simulink model "UUV_System"  (R2016a)
settings: Solver=VariableStepAuto  StartTime=0.0  StopTime=100  RelTol=1e-3
settings Model: Creator=Administrator  LastModifiedBy=Administrator

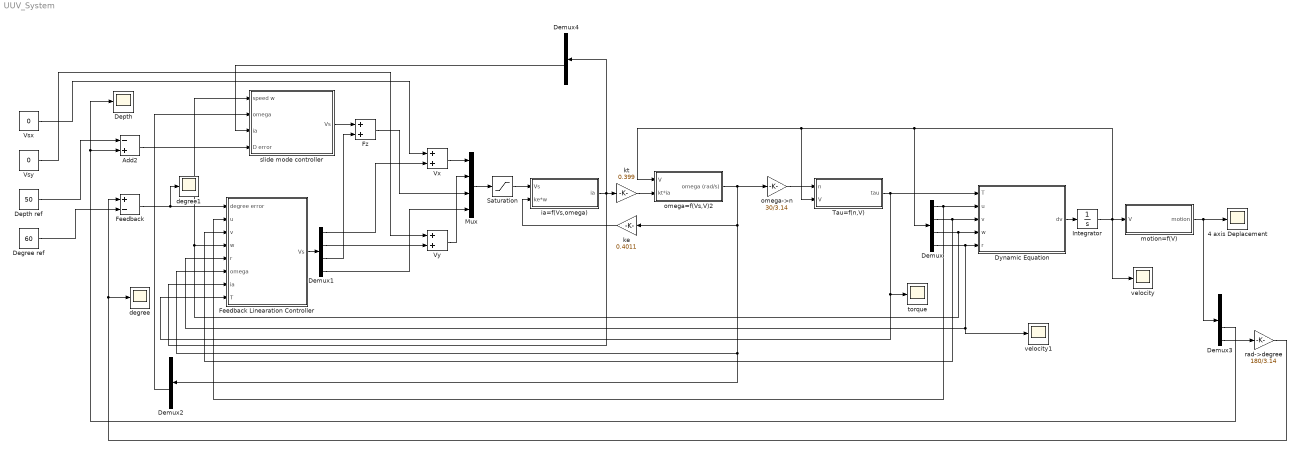
== system UUV_System ==
  "4 axis Deplacement " : Scope
  Add2 : Sum  Inputs=-+
  Degree ref : Constant  Value=60
  Demux{,1..4} (5 alike) : Demux
  Depth : Scope
  Depth ref : Constant  Value=50
  Dynamic Equation : MATLAB Function  TreatAsAtomicUnit=on
  Feedback : Sum  Inputs=+-
  Feedback Linearation Controller : Subsystem
  Fz : Sum
  Integrator : Integrator
  Mux : Mux
  Saturation : Saturate  UpperLimit=100  LowerLimit=-100
  Tau=f(n,V) : Subsystem
  Vsx : Constant  Value=0
  Vsy : Constant  Value=0
  Vx : Sum
  Vy : Sum
  degree : Scope
  degree1 : Scope
  ia=f(Vs,omega) : Subsystem
  ke : Gain  Gain=0.4011
  kt : Gain  Gain=0.399
  motion=f(V) : Subsystem
  omega->n : Gain  Gain=30/3.14
  omega=f(Vs,V)2 : Subsystem
  rad->degree : Gain  Gain=180/3.14
  slide mode controller : Subsystem
  torque : Scope
  velocity : Scope
  velocity1 : Scope
  wires:
  ia=f(Vs,omega)/1(ia) -> Feedback Linearation Controller/7(ia), Demux4/1, kt/1
  kt/1 -> omega=f(Vs,V)2/2(kt*ia)
  omega=f(Vs,V)2/1(omega (rad/s)) -> omega->n/1, Feedback Linearation Controller/6(omega), Demux2/1, ke/1
  ke/1 -> ia=f(Vs,omega)/2(ke*w)
  omega->n/1 -> Tau=f(n,V)/1(n)
  Tau=f(n,V)/1(tau) -> Dynamic Equation/1(T), Feedback Linearation Controller/8(T), torque/1
  Dynamic Equation/1(dv) -> Integrator/1
  Integrator/1 -> motion=f(V)/1(V), Demux/1, Tau=f(n,V)/2(V), omega=f(Vs,V)2/1(V), velocity/1
  Demux/1 -> Feedback Linearation Controller/2(u), Dynamic Equation/2(u)
  Demux/2 -> Feedback Linearation Controller/3(v), Dynamic Equation/3(v)
  Demux/3 -> Dynamic Equation/4(w), slide mode controller/1(speed w), Feedback Linearation Controller/4(w)
  Demux/4 -> velocity1/1, Feedback Linearation Controller/5(r), Dynamic Equation/5(r)
  motion=f(V)/1(motion) -> "4 axis Deplacement "/1, Demux3/1
  Demux1/4 -> Mux/4
  slide mode controller/1(Vs) -> Fz/1
  Demux1/3 -> Fz/2
  Fz/1 -> Mux/3
  Demux1/2 -> Vy/2
  Demux1/1 -> Vx/2
  Vx/1 -> Mux/1
  Vy/1 -> Mux/2
  Demux2/3 -> slide mode controller/2(omega)
  Degree ref/1 -> Feedback/2
  Feedback/1 -> degree1/1, Feedback Linearation Controller/1(degree error)
  Demux4/3 -> slide mode controller/3(ia)
  Depth ref/1 -> Add2/1
  Add2/1 -> slide mode controller/4(D error)
  Demux3/3 -> Depth/1, Add2/2
  Vsx/1 -> Vx/1
  Vsy/1 -> Vy/1
  Mux/1 -> Saturation/1
  Saturation/1 -> ia=f(Vs,omega)/1(Vs)
  Demux3/4 -> rad->degree/1
  rad->degree/1 -> degree/1, Feedback/1
  Feedback Linearation Controller/1(Vs) -> Demux1/1

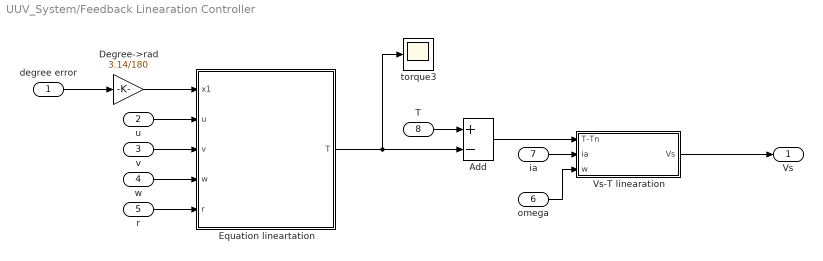
== system UUV_System/Feedback Linearation Controller ==
  degree error : Inport
  u : Inport  Port=2
  v : Inport  Port=3
  w : Inport  Port=4
  r : Inport  Port=5
  omega : Inport  Port=6
  ia : Inport  Port=7
  T : Inport  Port=8
  Add : Sum  Inputs=+-
  Degree->rad : Gain  Gain=3.14/180
  Equation lineartation : MATLAB Function  TreatAsAtomicUnit=on
  Vs-T linearation : Subsystem
  torque3 : Scope
  Vs : Outport
  wires:
  Vs-T linearation/1(Vs) -> Vs/1
  Add/1 -> Vs-T linearation/1(T-Tn)
  Equation lineartation/1(T) -> torque3/1, Add/2
  ia/1 -> Vs-T linearation/2(ia)
  omega/1 -> Vs-T linearation/3(w)
  T/1 -> Add/1
  u/1 -> Equation lineartation/2(u)
  r/1 -> Equation lineartation/5(r)
  w/1 -> Equation lineartation/4(w)
  v/1 -> Equation lineartation/3(v)
  Degree->rad/1 -> Equation lineartation/1(x1)
  degree error/1 -> Degree->rad/1

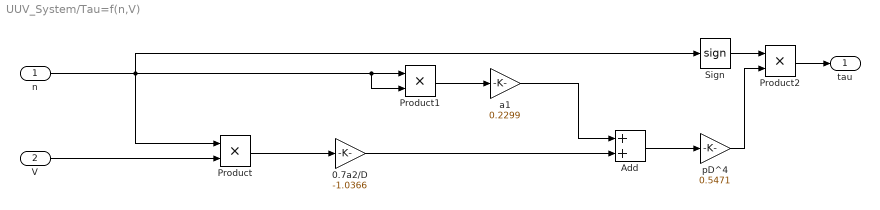
== system UUV_System/Tau=f(n,V) ==
  n : Inport
  V : Inport  Port=2
  0.7a2/D : Gain  Gain=-1.0366
  Add : Sum
  Product : Product
  Product1 : Product
  Product2 : Product
  Sign : Signum
  a1 : Gain  Gain=0.2299
  pD^4 : Gain  Gain=0.5471
  tau : Outport
  wires:
  n/1 -> Sign/1, Product/1, Product1/2, Product1/1
  V/1 -> Product/2
  Product1/1 -> a1/1
  Product/1 -> 0.7a2/D/1
  a1/1 -> Add/1
  0.7a2/D/1 -> Add/2
  Add/1 -> pD^4/1
  Sign/1 -> Product2/1
  pD^4/1 -> Product2/2
  Product2/1 -> tau/1

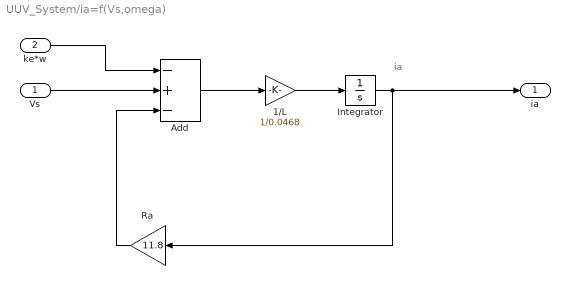
== system UUV_System/ia=f(Vs,omega) ==
  note: ia
  Vs : Inport
  ke*w : Inport  Port=2
  1/L : Gain  Gain=1/0.0468
  Add : Sum  Inputs=-+-
  Integrator : Integrator
  Ra : Gain  Gain=11.8
  ia : Outport
  wires:
  Add/1 -> 1/L/1
  1/L/1 -> Integrator/1
  Integrator/1 -> ia/1, Ra/1
  Ra/1 -> Add/3
  Vs/1 -> Add/2
  ke*w/1 -> Add/1

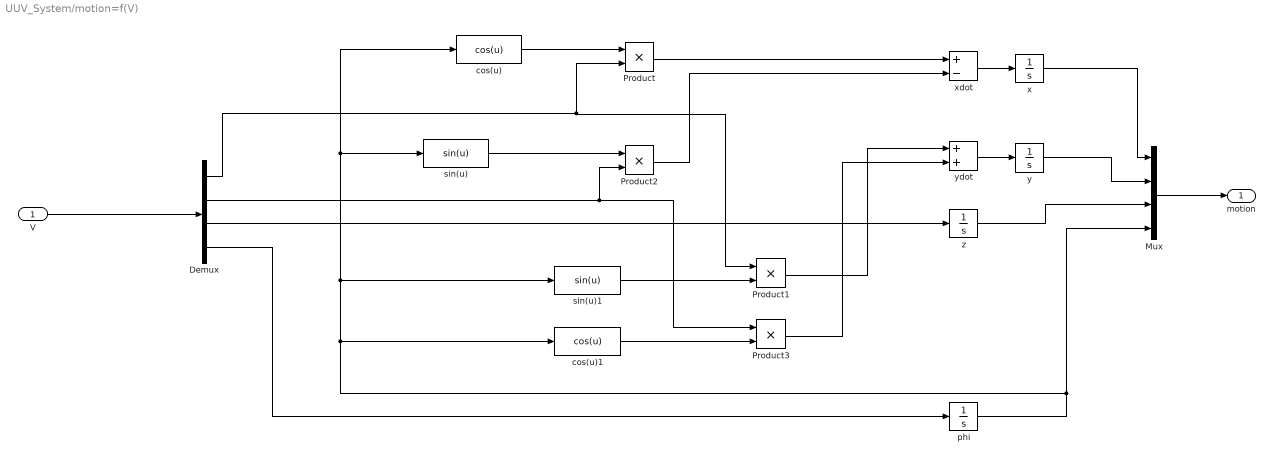
== system UUV_System/motion=f(V) ==
  V : Inport
  Demux : Demux
  Mux : Mux
  Product{,1..3} (4 alike) : Product
  cos(u) : MATLABFcn  MATLABFcn=cos(u)
  cos(u)1 : MATLABFcn  MATLABFcn=cos(u)
  phi : Integrator
  sin(u) : MATLABFcn  MATLABFcn=sin(u)
  sin(u)1 : MATLABFcn  MATLABFcn=sin(u)
  x : Integrator
  xdot : Sum  Inputs=+-
  y : Integrator
  ydot : Sum
  z : Integrator
  motion : Outport
  wires:
  V/1 -> Demux/1
  cos(u)/1 -> Product/1
  Demux/1 -> Product/2, Product1/1
  Product/1 -> xdot/1
  sin(u)/1 -> Product2/1
  Demux/2 -> Product3/1, Product2/2
  Product2/1 -> xdot/2
  sin(u)1/1 -> Product1/2
  cos(u)1/1 -> Product3/2
  Product1/1 -> ydot/1
  Product3/1 -> ydot/2
  Demux/3 -> z/1
  Demux/4 -> phi/1
  z/1 -> Mux/3
  Mux/1 -> motion/1
  phi/1 -> Mux/4, cos(u)1/1, sin(u)1/1, cos(u)/1, sin(u)/1
  xdot/1 -> x/1
  x/1 -> Mux/1
  ydot/1 -> y/1
  y/1 -> Mux/2

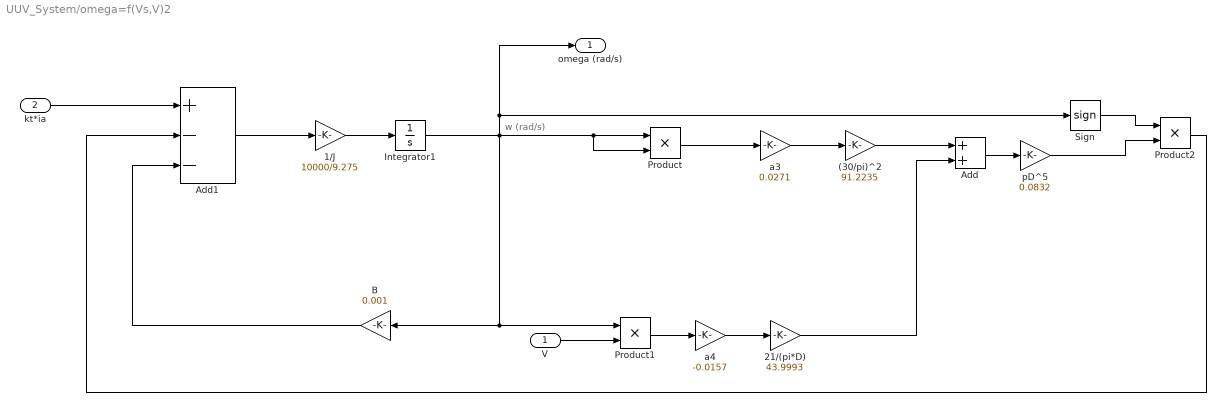
== system UUV_System/omega=f(Vs,V)2 ==
  note: w (rad/s)
  V : Inport
  kt*ia : Inport  Port=2
  (30/pi)^2 : Gain  Gain=91.2235
  1/J : Gain  Gain=10000/9.275
  21/(pi*D) : Gain  Gain=43.9993
  Add : Sum
  Add1 : Sum  Inputs=+--
  B : Gain  Gain=0.001
  Integrator1 : Integrator
  Product : Product
  Product1 : Product
  Product2 : Product
  Sign : Signum
  a3 : Gain  Gain=0.0271
  a4 : Gain  Gain=-0.0157
  pD^5 : Gain  Gain=0.0832
  omega (rad/s) : Outport
  wires:
  1/J/1 -> Integrator1/1
  Add1/1 -> 1/J/1
  B/1 -> Add1/3
  Integrator1/1 -> Product/2, Product/1, omega (rad/s)/1, Sign/1, Product1/1, B/1
  kt*ia/1 -> Add1/1
  Product/1 -> a3/1
  a3/1 -> (30/pi)^2/1
  (30/pi)^2/1 -> Add/1
  a4/1 -> 21/(pi*D)/1
  V/1 -> Product1/2
  Product1/1 -> a4/1
  21/(pi*D)/1 -> Add/2
  Add/1 -> pD^5/1
  Sign/1 -> Product2/1
  pD^5/1 -> Product2/2
  Product2/1 -> Add1/2

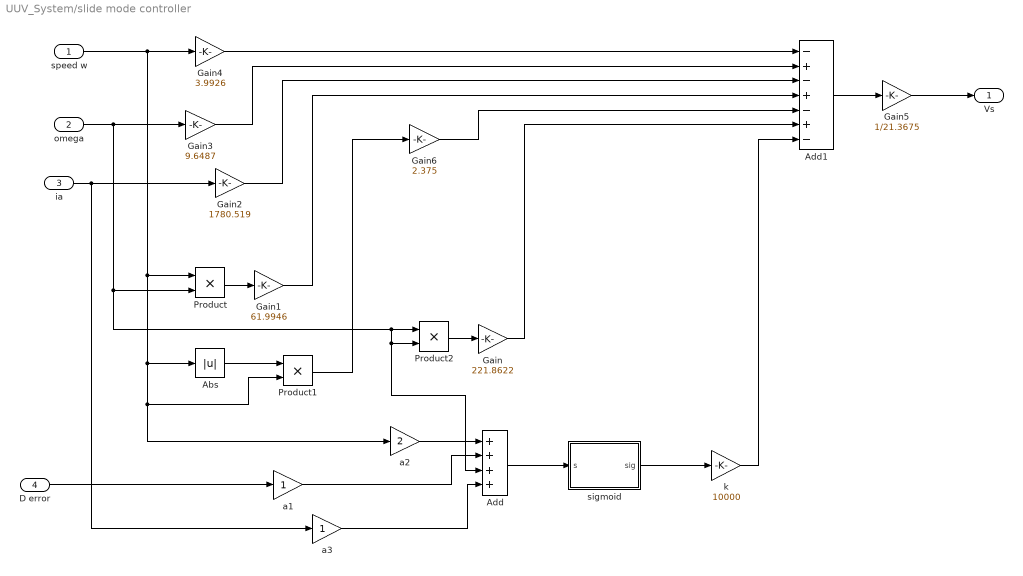
== system UUV_System/slide mode controller ==
  speed w : Inport
  omega : Inport  Port=2
  ia : Inport  Port=3
  D error : Inport  Port=4
  Abs : Abs
  Add : Sum  Inputs=++++
  Add1 : Sum  Inputs=-+-+-+-
  Gain : Gain  Gain=221.8622
  Gain1 : Gain  Gain=61.9946
  Gain2 : Gain  Gain=1780.519
  Gain3 : Gain  Gain=9.6487
  Gain4 : Gain  Gain=3.9926
  Gain5 : Gain  Gain=1/21.3675
  Gain6 : Gain  Gain=2.375
  Product : Product
  Product1 : Product
  Product2 : Product
  a1 : Gain
  a2 : Gain  Gain=2
  a3 : Gain
  k : Gain  Gain=10000
  sigmoid : MATLAB Function  TreatAsAtomicUnit=on
  Vs : Outport
  wires:
  speed w/1 -> a2/1, Product1/2, Abs/1, Product/1, Gain4/1
  omega/1 -> Add/3, Product2/2, Product2/1, Product/2, Gain3/1
  ia/1 -> a3/1, Gain2/1
  Product/1 -> Gain1/1
  Gain4/1 -> Add1/1
  Gain3/1 -> Add1/2
  Gain2/1 -> Add1/3
  Gain1/1 -> Add1/4
  Abs/1 -> Product1/1
  Product2/1 -> Gain/1
  Gain/1 -> Add1/6
  D error/1 -> a1/1
  a2/1 -> Add/1
  a1/1 -> Add/2
  k/1 -> Add1/7
  Add1/1 -> Gain5/1
  Gain5/1 -> Vs/1
  a3/1 -> Add/4
  Add/1 -> sigmoid/1(s)
  Gain6/1 -> Add1/5
  Product1/1 -> Gain6/1
  sigmoid/1(sig) -> k/1

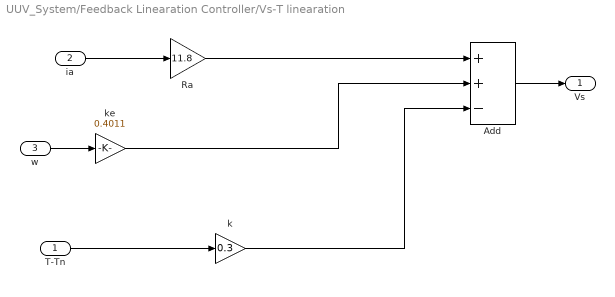
== system UUV_System/Feedback Linearation Controller/Vs-T linearation ==
  T-Tn : Inport
  ia : Inport  Port=2
  w : Inport  Port=3
  Add : Sum  Inputs=++-
  Ra : Gain  Gain=11.8
  k : Gain  Gain=0.3
  ke : Gain  Gain=0.4011
  Vs : Outport
  wires:
  ia/1 -> Ra/1
  Ra/1 -> Add/1
  w/1 -> ke/1
  ke/1 -> Add/2
  Add/1 -> Vs/1
  T-Tn/1 -> k/1
  k/1 -> Add/3

== matlab function UUV_System/Dynamic Equation ==
  data: T input; dv output; u input; v input; w input; r input
function dv = fcn(T,u,v,w,r)
%#codegen

%%velocity
vel=[u;v;w;r];
%% propeller
D=0.152;

%% motor
J=9.275*1e-4;
ke=0.4011;
Ra=11.8;
L=0.0468;
kt=0.399;
B=0.001;
m=128;
g=9.8;

%%cordinate
xG=0;yG=0;zG=0.054;
Iz=14.213;

%%matirx
Mrb=[m 0 0 -m*yG;0 m 0 m*xG;0 0 m 0;-m*yG m*xG 0 Iz];
Ma=-1*[-33.48 0 0 0;0 -110.8941 0 -4.921;0 0 -147.576 0;0 -4.921 0 -12.75];
Crb=-1*[0 0 0 -m*(xG*r+v);0 0 0 -m*(yG*r-u);0 0 0 0;m*(xG*r+v) m*(yG*r-u) 0 0];
Ca=-1*[0 0 0 -110.8941*v-4.921*r;0 0 0 33.48*u;0 0 0 0;110.8941*v+4.921*r -33.48*u 0 0];
Dv=-1*[-4.9217-139.8007*abs(u) 0 0 0;0 -3.0591-350.2618*abs(v) 0 0;0 0 -4.4132-327.2375*abs(w) 0;0 0 0 -1.3881-51.1709*abs(r)];
G=[0;0;0;0];

%% Equation
tau=T;

dvel=(Mrb+Ma)^(-1)*(tau-G-(Crb+Ca+Dv)*vel);  %% state equation

%%output
dv=dvel;

== matlab function UUV_System/slide mode controller/sigmoid ==
  data: s input; sig output
function sig = fcn(s)
%#codegen
if s<=-1
    u=-1;
else if s>-1&&s<=1
        u=s;
    else
        u=1;
    end
end        

sig = u;

== matlab function UUV_System/Feedback Linearation Controller/Equation lineartation ==
  data: x1 input; u input; v input; w input; T output; r input
function T = fcn(x1,u,v,w,r)
%#codegen

%%velocity
vel=[u;v;w;r];
%% propeller
D=0.152;

%% motor
J=9.275*1e-4;
ke=0.4011;
Ra=11.8;
L=0.0468;
kt=0.399;
B=0.001;
m=128;
g=9.8;

%%cordinate
xG=0;yG=0;zG=0.054;
Iz=14.213;

%%matirx
Mrb=[m 0 0 -m*yG;0 m 0 m*xG;0 0 m 0;-m*yG m*xG 0 Iz];
Ma=-1*[-33.48 0 0 0;0 -110.8941 0 -4.921;0 0 -147.576 0;0 -4.921 0 -12.75];
Crb=-1*[0 0 0 -m*(xG*r+v);0 0 0 -m*(yG*r-u);0 0 0 0;m*(xG*r+v) m*(yG*r-u) 0 0];
Ca=-1*[0 0 0 -110.8941*v-4.921*r;0 0 0 33.48*u;0 0 0 0;110.8941*v+4.921*r -33.48*u 0 0];
Dv=-1*[-4.9217-139.8007*abs(u) 0 0 0;0 -3.0591-350.2618*abs(v) 0 0;0 0 -4.4132-327.2375*abs(w) 0;0 0 0 -1.3881-51.1709*abs(r)];
G=[0;0;0;0];


%% Lineartion
N=Crb+Ca+Dv;
A=Mrb+Ma;

Mz=A*[u;v;w;-0.3*x1-1*r]; %% pole configuration
a=N*vel;

a(4)+Mz(4); %%Choose Mz as U,then linearize

%%output
T=[0;0;0;a(4)+Mz(4)];
